simulink model "fitdf2filter_demo"  (Simulink 7.6)
settings: Solver=FixedStepDiscrete  StartTime=0.0  StopTime=n(end)  RelTol=1e-3
InitFcn:
  | ;
StartFcn:
  | ;
StopFcn:
  | ;
PreSaveFcn:
  | ;
CloseFcn:
  | ;
settings Model: Creator=tbryan  LastModifiedBy=vsriniva  ExtModeAutoUpdateStatusClock=off
settings DataIOCC: SignalLoggingName=logsOut
settings OptimizationCC: InlineInvariantSignals=on  InitFltsAndDblsToZero=on
settings DebuggingCC: SaveWithParameterizedLinksMsg=none  CheckExecutionContextPreStartOutputMsg=on  CheckExecutionContextRuntimeOutputMsg=on  SignalResolutionControl=TryResolveAllWithWarning  MultiTaskDSMMsg=warning  MultiTaskCondExecSysMsg=none  ParameterDowncastMsg=none  ParameterOverflowMsg=none  ParameterPrecisionLossMsg=none  StrictBusMsg=None
settings HardwareCC: ProdHWDeviceType=ASIC/FPGA->ASIC/FPGA  TargetBitPerLong=64  TargetEndianess=LittleEndian  TargetWordSize=64  TargetHWDeviceType=MATLAB Host  ProdEqTarget=off
settings RTWCC: IncludeERTFirstTime=on
settings GRTTargetCC: TargetFcnLib=ansi_tfl_tmw.mat

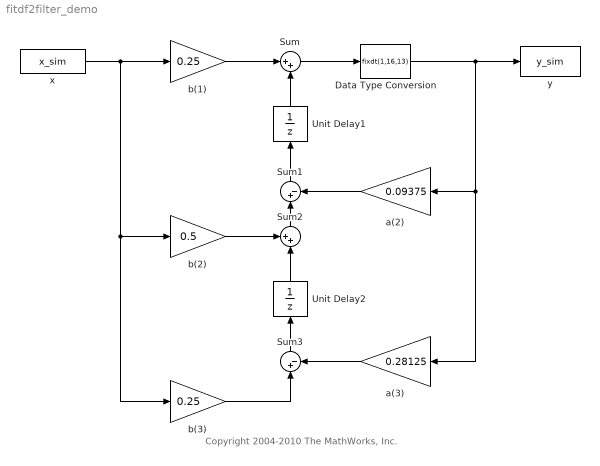
== system fitdf2filter_demo ==
  note: Copyright 2004-2010 The MathWorks, Inc.
  Data Type Conversion : DataTypeConversion  OutDataTypeMode=Specify via dialog  OutDataType=fixdt(1,16,13)  OutDataTypeStr=fixdt(1,16,13)  RndMeth=Nearest  SaturateOnIntegerOverflow=on  LockScale=on
  Sum : Sum  Inputs=|++  OutDataType=sfix(8)  OutScaling=2^-6  RndMeth=Nearest  SaturateOnIntegerOverflow=on
  Sum1 : Sum  Inputs=|+-  OutDataTypeMode=Specify via dialog  OutDataType=fixdt(1,16,14)  OutDataTypeStr=fixdt(1,16,14)  RndMeth=Nearest  SaturateOnIntegerOverflow=on
  Sum2 : Sum  Inputs=++|  OutDataType=sfix(16)  OutScaling=2^0  RndMeth=Nearest  SaturateOnIntegerOverflow=on
  Sum3 : Sum  Inputs=|+-  OutDataTypeMode=Specify via dialog  OutDataType=fixdt(1,16,14)  OutDataTypeStr=fixdt(1,16,14)  RndMeth=Nearest  SaturateOnIntegerOverflow=on
  Unit Delay1 : UnitDelay
  Unit Delay2 : UnitDelay
  a(2) : Gain  Gain=0.09375  ParameterDataTypeMode=Specify via dialog  ParameterDataType=fixdt(1,8,6)  ParamDataTypeStr=fixdt(1,8,6)  OutDataType=sfix(16)  OutScaling=2^0  RndMeth=Nearest  SaturateOnIntegerOverflow=on
  a(3) : Gain  Gain=0.28125  ParameterDataTypeMode=Specify via dialog  ParameterDataType=fixdt(1,8,6)  ParamDataTypeStr=fixdt(1,8,6)  OutDataType=sfix(16)  OutScaling=2^0  RndMeth=Nearest  SaturateOnIntegerOverflow=on
  b(1) : Gain  Gain=0.25  ParameterDataTypeMode=Specify via dialog  ParameterDataType=fixdt(1,8,6)  ParamDataTypeStr=fixdt(1,8,6)  OutDataType=sfix(16)  OutScaling=2^0  RndMeth=Nearest  SaturateOnIntegerOverflow=on
  b(2) : Gain  Gain=0.5  ParameterDataTypeMode=Specify via dialog  ParameterDataType=fixdt(1,8,6)  ParamDataTypeStr=fixdt(1,8,6)  OutDataType=sfix(16)  OutScaling=2^0  RndMeth=Nearest  SaturateOnIntegerOverflow=on
  b(3) : Gain  Gain=0.25  ParameterDataTypeMode=Specify via dialog  ParameterDataType=fixdt(1,8,6)  ParamDataTypeStr=fixdt(1,8,6)  OutDataType=sfix(16)  OutScaling=2^0  RndMeth=Nearest  SaturateOnIntegerOverflow=on
  x : FromWorkspace  VariableName=x_sim  SampleTime=0  Interpolate=off  OutputAfterFinalValue=Setting to zero
  y : ToWorkspace  VariableName=y_sim  SampleTime=-1  SaveFormat=Array
  wires:
  a(2)/1 -> Sum1/2
  b(2)/1 -> Sum2/1
  a(3)/1 -> Sum3/2
  Sum3/1 -> Unit Delay2/1
  Sum2/1 -> Sum1/1
  b(1)/1 -> Sum/1
  Unit Delay1/1 -> Sum/2
  x/1 -> b(2)/1, b(3)/1, b(1)/1
  Sum/1 -> Data Type Conversion/1
  b(3)/1 -> Sum3/1
  Data Type Conversion/1 -> y/1, a(3)/1, a(2)/1
  Unit Delay2/1 -> Sum2/2
  Sum1/1 -> Unit Delay1/1
